simulink model "TfContinuousModel_OptimalControlIntegral_Obs_mdl"  (Simulink 7.5)
settings: Solver=ode45  StartTime=0.0  StopTime=10.0  FixedStep=Ts  RelTol=1e-3
values from neighbouring files (symbols this model uses):
  H = Ki(n+1)    [TSC150715ProvaMatlab.m]
  K = Ki(1:n)    [TSC150715ProvaMatlab.m]
  L = -acker(Az',Cz',[0 0 0])'    [TSC150715ProvaMatlab.m]
  Ts = 0.01    [TSC150715ProvaMatlab.m]
  yp = 12    [TSC150715ProvaMatlab.m]
undefined symbols (not defined in the file or in its folder): Az, Bz, Cz, DiscIntNeverNeededParam
libraries: cstblocks x1
settings Model: Creator=lbiagiotti  LastModifiedBy=Biagio
settings DebuggingCC: SaveWithParameterizedLinksMsg=none  MultiTaskDSMMsg=warning  MultiTaskCondExecSysMsg=none  StrictBusMsg=None
settings HardwareCC: TargetHWDeviceType=32-bit Generic
settings RTWCC: IncludeERTFirstTime=on
settings CodeAppCC: CustomSymbolStrType=$N$R$M_T
settings GRTTargetCC: TargetFcnLib=ansi_tfl_tmw.mat

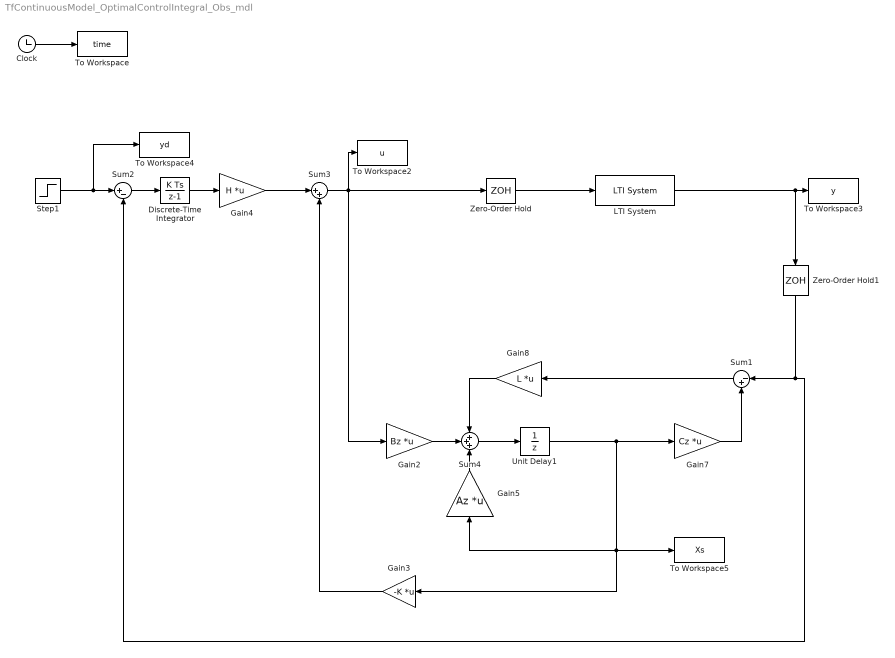
== system TfContinuousModel_OptimalControlIntegral_Obs_mdl ==
  Clock : Clock
      settings: Decimation=10
  Discrete-Time Integrator : DiscreteIntegrator  SampleTime=Ts  ICPrevOutput=DiscIntNeverNeededParam  ICPrevScaledInput=DiscIntNeverNeededParam
  Gain2 : Gain  Gain=Bz  Multiplication=Matrix(K*u)
  Gain3 : Gain  Gain=-K  Multiplication=Matrix(K*u)
  Gain4 : Gain  Gain=H  Multiplication=Matrix(K*u)
  Gain5 : Gain  Gain=Az  Multiplication=Matrix(K*u)
  Gain7 : Gain  Gain=Cz  Multiplication=Matrix(K*u)
  Gain8 : Gain  Gain=L  Multiplication=Matrix(K*u)
  LTI System : cstblocks/LTI System  SystemSampleTime=-1  sys=G  IC=[]
  Step1 : Step  After=yp  SampleTime=0
  Sum1 : Sum  Inputs=|-+
  Sum2 : Sum  Inputs=|+-
  Sum3 : Sum  Inputs=|++
  Sum4 : Sum  Inputs=+++
  To Workspace : ToWorkspace  VariableName=time  SampleTime=-1  SaveFormat=Array
  To Workspace2 : ToWorkspace  VariableName=u  SampleTime=-1  SaveFormat=Array
  To Workspace3 : ToWorkspace  VariableName=y  SampleTime=-1  SaveFormat=Array
  To Workspace4 : ToWorkspace  VariableName=yd  SampleTime=-1  SaveFormat=Array
  To Workspace5 : ToWorkspace  VariableName=Xs  SampleTime=-1  SaveFormat=Array
  Unit Delay1 : UnitDelay  SampleTime=Ts
  Zero-Order Hold : ZeroOrderHold  SampleTime=Ts
  Zero-Order Hold1 : ZeroOrderHold  SampleTime=Ts
  wires:
  Step1/1 -> To Workspace4/1, Sum2/1
  Clock/1 -> To Workspace/1
  Discrete-Time Integrator/1 -> Gain4/1
  Sum2/1 -> Discrete-Time Integrator/1
  Gain3/1 -> Sum3/2
  Sum3/1 -> To Workspace2/1, Gain2/1, Zero-Order Hold/1
  Gain4/1 -> Sum3/1
  LTI System/1 -> To Workspace3/1, Zero-Order Hold1/1
  Sum4/1 -> Unit Delay1/1
  Unit Delay1/1 -> Gain7/1, Gain3/1, To Workspace5/1, Gain5/1
  Gain2/1 -> Sum4/2
  Gain5/1 -> Sum4/3
  Gain8/1 -> Sum4/1
  Sum1/1 -> Gain8/1
  Gain7/1 -> Sum1/2
  Zero-Order Hold/1 -> LTI System/1
  Zero-Order Hold1/1 -> Sum2/2, Sum1/1
